simulink model "HIL_Testing_SW_amantest"  (Simulink 7.5)
settings: Solver=ode1  StartTime=0.0  StopTime=Inf  FixedStep=0.001  RelTol=1e-3
PostLoadFcn:
  | , if any(exist('dsrtsu_mdlpostloadfcn', 'file') == [2, 3, 6]), try dsrtsu_mdlpostloadfcn('Execute', bdroot); catch fprintf('Error in PostLoadFcn (dsrtsu_mdlpostloadfcn) for model "%s":\n %s\n', bdroot, lasterr); end, end,
undefined symbols (not defined in the file): CeBSER_Cnt_NumTempAxisPts, ChargeCord, ChargeCord_Control, ChargeToSOCCurr, ChrgCurrLim, CrntSens1Fine, CS_SOCSetPt, CyclerMaxChrgPwr, CyclerMaxDschrgPwr, deltaAhr, Drive_1, Drive_10, Drive_11, Drive_12, Drive_13, Drive_14, Drive_15, Drive_16, Drive_17, Drive_18, Drive_19, Drive_2, Drive_20, Drive_21, Drive_22, Drive_23, Drive_24, Drive_25, Drive_26, Drive_27, Drive_28, Drive_29, Drive_3, Drive_30, Drive_31, Drive_32, Drive_33, Drive_34, Drive_35, Drive_36, Drive_37, Drive_38, Drive_39, Drive_4, Drive_40, Drive_41, Drive_42, Drive_43, Drive_44, Drive_45, Drive_46, Drive_47, Drive_48, Drive_49, Drive_5, Drive_50, Drive_51, Drive_6, Drive_7, Drive_8 ... (+50)
libraries: simulink x129, rtican x50, rti2211sailib x5, rti2211serlib x5, rti2202miolib x3
(part 6 of 23)

== system HIL_Testing_SW_amantest/HWO/TX HVEM/msg_Charge ==
  note: unsure about this one
  HVCD_ACInputVltg : Inport  OutDataType=fixdt(1, 16)  OutScaling=2^0
  HVCD_ACInputCurr : Inport  Port=2  OutDataType=fixdt(1, 16)  OutScaling=2^0
  HVCD_ACInputTemp : Inport  Port=3  OutDataType=fixdt(1, 16)  OutScaling=2^0
  Current : Inport  Port=4  OutDataType=sfix(16)  OutScaling=2^0
  Voltage : Inport  Port=5  OutDataType=fixdt(1, 16)  OutScaling=2^0
  Trigger : TriggerPort  TriggerType=function-call
  ACInputCrntV{,1..3} (4 alike) : Constant  Value=0  OutDataTypeMode=double  OutDataType=fixdt(1, 16)  OutScaling=2^0  OutDataTypeStr=double
  ChargeFlashStat : Constant  Value=0  OutDataType=fixdt(1, 16)  OutScaling=2^0
  ChrgReadStat2 : Constant  Value=20  OutDataType=fixdt(1, 16)  OutScaling=2^0
  ChrgReadStat3 : Constant  Value=200  OutDataType=fixdt(1, 16)  OutScaling=2^0
  ChrgrPmpPrcntSpd : Constant  Value=0  OutDataType=fixdt(1, 16)  OutScaling=2^0
  HVChrgLV{,1..4} (5 alike) : Constant  OutDataType=fixdt(1, 16)  OutScaling=2^0
  High_Voltage_Charger_Data_HV : rtican/RTICAN Transmit (TX)   SystemSampleTime=-1  Reserved1=[]  Reserved2=[]  Reserved3=[]  Reserved4=[]  SfcnMessage=[]  Msg_Struct=[]  BoardTypeNo=[]  BoardNo=[]  ChannelNo=[]  Parameters=[]  DialogFcn=[]  UnitName=[]  Revision=[]  UnitValues=[]  DSProperties=struct('RTI',struct('Version',uint32(5),'BlockType',struct('isSLSource',uint8(1),'isSLSink',uint8(1),'isHWSource',uint8(0),'isHWSink',uint8(0),'isSetup',uint8(0),'isInline',uint8(1),'isNonInline',uint8(0),'isInterrupt',uint8(0),'isChannelwise',uint8(0)),'IOBoardType','RTICAN','UnitType','MESSAGE','Identifier','TX','DialogType','MSVC','BlockSet','RTICAN','SlaveProcessor','CAN'))  RTIBlockInterface=struct('InputPortsWidth',int32([1 1 1 1 1 1 1 1 1]),'InputPortsActive',[1 1 1 1 1 1 1 1 1],'InputPortsName',{{'HVChrgRdnsStat','HVCD_ChgrFlshStat','HVCD_Tmp','HVCD_ACInptVltg','HVCD_ACInptCrnt','HVCD_ACInptCrntV','HVCD_ACInptVltgV','HVCD_TmpV','HVChgrActDisStat'}},'InputPortsDataType',{{'SS_DOUBLE','SS_DOUBLE','SS_DOUBLE','SS_DOUBLE','SS_DOUBLE','SS_DOUBLE','SS_DOUBLE','SS_DOUBLE','SS_DOUBLE'}},'OutputPortsWidth',int32(1),'OutputPortsActive',1,'OutputPortsName',{{['TX status']}},'DialogFcn','rtican_message_interface_gui','BlockDisplay',{{'','center'}},'IconTransparency','on','InitLevel',3,'BlockName',struct('Token',{{'High_Voltage_Charger_Data_HV'}}),'SampleTime',{{-1}},'TriggerPort',{{'none'}},'EnablePort',{{'none'}})  RTIBlockParameters=struct('BoardTypeNo',{{4302,'OFF',[]}},'BoardNo',{{1,'ON',[1 16]}},'ChannelNo',{{4,'ON',[1 4]}},'Parameters',{{struct('DataFileSupport',struct('DataFileSelectedMaster',1,'DataFileSelectedLocal',1,'DataFileName',['c:\data\databases\8.0.1 (13015)\globala - hv.dbc|c:\data\testing\dbc\globala - hvdmx112.dbc|'],'DataFileDate',{{{['04-Jan-2013 08:37:04']},{['10-May-2011 15:46:00']}}},'SelectedFile',['..\databases\8.0.1 (13015)\globala - hv.dbc'],'InterfaceFcn','rtican_dbc_file_parser'),'Options',struct('StatusSelected',1,'TimeSelected',0,'DeltaTimeSelected',0,'DelayTimeSelected',0,'DelayTimeTXCommandSelected',0,'EncodeSetUnusedBitsToOne',0,'EnableMsgLoopback',0,'TriggerPort',struct('Selected',0,'TriggerType',0),'EnablePortSelected',0,'SignalOnPortnameSelected',1,'UserCoding',struct('Selected',0,'InterfaceFile','UserEncodingFile','FcnName','UserEncodeFcn','InportSelected',0,'InportWidth',1,'OutportSelected',0,'OutportWidth',1),'TerminationMsg',struct('Selected',0,'Byte0_7','0'),'InitialMsg',struct('Selected',0,'Byte0_7','0')),'Message',struct('MsgOnBlocknameSelected',1,'MsgName','High_Voltage_Charger_Data_HV','MsgIdFormat',0,'MsgId',778,'MsgLength',7,'NumSignals',9,'SampleTime',-1,'StartTime',struct('Selected',0,'Value',0),'AutoRepeatTime',struct('Selected',0,'Value',0.1),'Timeout',struct('Selected',0,'Value',0.1),'DelayTime',struct('Selected',0,'Value',0.1),'Signal',struct('SgnName',{'HVChrgRdnsStat','HVCD_ChgrFlshStat','HVCD_Tmp','HVCD_ACInptVltg','HVCD_ACInptCrnt','HVCD_ACInptCrntV','HVCD_ACInptVltgV','HVCD_TmpV','HVChgrActDisStat'},'SgnStartBit',{25,27,28,36,44,52,53,54,55},'SgnLength',{2,1,8,8,8,1,1,1,1},'SgnType',{0,0,0,0,0,0,0,0,0},'ModeValue',{-1,-1,-1,-1,-1,-1,-1,-1,-1},'DataType',{0,0,0,0,0,0,0,0,0},'ByteLayout',{2,2,2,2,2,2,2,2,2},'Factor',{1,1,0.5,2,0.2,1,1,1,1},'Offset',{0,0,-40,0,0,0,0,0,0},'SgnComment',{{''},{''},{''},{''},{''},{''},{''},{''},{''}},'SgnUnit',{'','',['deg C'],'V','A','','','',''},'Min',{0,0,-40,0,0,0,0,0,0},'Max',{3,1,87.5,510,51,1,1,1,1},'SLDataType',{'SS_DOUBLE','SS_DOUBLE','SS_DOUBLE','SS_DOUBLE','SS_DOUBLE','SS_DOUBLE','SS_DOUBLE','SS_DOUBLE','SS_DOUBLE'}),'MsgIdNumFormat',0,'MsgComment',{{''}}),'Version',1.2,'general',struct('isFromLib',0)),'OFF',[]}},'GroupId',{{struct('Group',{{'RTICAN'}},'No',7,'Behavior',{{'NAMECHANGE'}},'BlockType',{{'SINK'}},'NameChangeFlag',0),'OFF',[]}},'SFcnRTICANMessage',{{struct('MsgType','TX','SFcnPortType','Scalar','MsgName','High_Voltage_Charger_Data_HV','MsgIdFormat','STD','MsgId',778,'MsgLength',7,'NumSignals',9,'SampleTime',-1,'StartTime',struct('Selected','no','Value',0),'AutoRepeatTime',struct('Selected','no','Value',0.1),'Timeout',struct('Selected','no','Value',0.1),'Signal',struct('SgnName',{'HVChrgRdnsStat','HVCD_ChgrFlshStat','HVCD_Tmp','HVCD_ACInptVltg','HVCD_ACInptCrnt','HVCD_ACInptCrntV','HVCD_ACInptVltgV','HVCD_TmpV','HVChgrActDisStat'},'SgnStartBit',{25,27,28,36,44,52,53,54,55},'SgnLength',{2,1,8,8,8,1,1,1,1},'SgnType',{'standard','standard','standard','standard','standard','standard','standard','standard','standard'},'ModeValue',{-1,-1,-1,-1,-1,-1,-1,-1,-1},'DataType',{['unsigned int'],['unsigned int'],['unsigned int'],['unsigned int'],['unsigned int'],['unsigned int'],['unsigned int'],['unsigned int'],['unsigned int']},'ByteLayout',{['motorola back.'],['motorola back.'],['motorola back.'],['motorola back.'],['motorola back.'],['motorola back.'],['motorola back.'],['motorola back.'],['motorola back.']},'Factor',{1,1,0.5,2,0.2,1,1,1,1},'Offset',{0,0,-40,0,0,0,0,0,0},'SLDataType',{'SS_DOUBLE','SS_DOUBLE','SS_DOUBLE','SS_DOUBLE','SS_DOUBLE','SS_DOUBLE','SS_DOUBLE','SS_DOUBLE','SS_DOUBLE'}),'StatusSelected','yes','TimeSelected','no','DeltaTimeSelected','no','DelayTimeSelected','no','DelayTimeTXCommandSelected','no','EncodeSetUnusedBitsToOne','no','EnableMsgLoopback','no','TriggerPort',struct('Selected','no','TriggerType',0),'EnablePortSelected','no','UserCoding',struct('Selected','no','InterfaceFile','UserEncodingFile','FcnName','UserEncodeFcn','InportSelected','no','InportWidth',1,'OutportSelected','no','OutportWidth',1),'TerminationMsg',struct('Selected','no','Byte0','0x00','Byte1','0x00','Byte2','0x00','Byte3','0x00','Byte4','0x00','Byte5','0x00','Byte6','0x00','Byte7','0x00'),'InitialMsg',struct('Selected','no','Byte0','0x00','Byte1','0x00','Byte2','0x00','Byte3','0x00','Byte4','0x00','Byte5','0x00','Byte6','0x00','Byte7','0x00'),'BoardType','DS4302','BoardNo',1,'ControllerNo',4),'OFF',[]}},'TLCFileName',{{'rtican_tx_message','OFF',[]}})  RTISFcnParameters=struct('SFcnRTICANMessage','struct','TLCFileName','char')  RTIBlockParaDefault=struct('BoardTypeNo',4302,'BoardNo',1,'ChannelNo',1,'Parameters',struct('DataFileSupport',struct('DataFileSelectedMaster',0,'DataFileSelectedLocal',0,'DataFileName','','DataFileDate','','SelectedFile',['<no file selected>']),'Options',struct('StatusSelected',1,'TimeSelected',1,'DeltaTimeSelected',1,'DelayTimeSelected',1,'DelayTimeTXCommandSelected',0,'EncodeSetUnusedBitsToOne',0,'EnableMsgLoopback',0,'TriggerPort',struct('Selected',0,'TriggerType','rising'),'EnablePortSelected',0,'SignalOnPortnameSelected',1,'UserCoding',struct('Selected',0,'InterfaceFile','UserEncodingFile','FcnName','UserEncodeFcn','InportSelected',0,'InportWidth',1,'OutportSelected',0,'OutportWidth',1),'TerminationMsg',struct('Selected',0,'Byte0_7','0'),'InitialMsg',struct('Selected',0,'Byte0_7','0')),'Message',struct('MsgOnBlocknameSelected',0,'MsgName',['TX Message'],'MsgIdFormat',0,'MsgId',100,'MsgLength',8,'NumSignals',1,'SampleTime',-1,'StartTime',struct('Selected',0,'Value',0),'AutoRepeatTime',struct('Selected',0,'Value',0.1),'Timeout',struct('Selected',0,'Value',0.1),'DelayTime',struct('Selected',0,'Value',0.1),'Signal',struct('SgnName',['TX signal'],'SgnStartBit',0,'SgnLength',8,'SgnType',0,'ModeValue',-1,'DataType',0,'SLDataType','SS_DOUBLE','ByteLayout',0,'Factor',1,'Offset',0,'Min',0,'Max',255,'SgnComment',{{}},'SgnUnit',''),'MsgIdNumFormat',0,'MsgComment',{{''}}),'Version',1.2,'general',struct('isFromLib',1)),'GroupId',struct('Group',{{'RTICAN'}},'No',1,'Behavior',{{'NAMECHANGE'}},'BlockType',{{'SINK'}},'NameChangeFlag',0),'SFcnRTICANMessage',struct('MsgType','TX','MsgName',['TX Message'],'MsgIdFormat','STD','MsgId',100,'MsgLength',2,'NumSignals',1,'SampleTime',-1,'StartTime',struct('Selected','no','Value',0),'AutoRepeatTime',struct('Selected','no','Value',0.1),'Timeout',struct('Selected','no','Value',0.1),'DelayTime',struct('Selected','no','Value',0.1),'Signal',struct('SgnName',['TX signal'],'SgnStartBit',0,'SgnLength',8,'SgnType','standard','ModeValue',-1,'DataType',['unsigned int'],'ByteLayout',['little endian'],'SLDataType','SS_DOUBLE','Factor',1,'Offset',0),'StatusSelected','yes','TimeSelected','yes','DeltaTimeSelected','yes','DelayTimeSelected','yes','EnablePortSelected','no','EnableMsgLoopback','no','DelayTimeTXCommandSelected','no','EncodeSetUnusedBitsToOne','no','UserCoding',struct('Selected','no','InterfaceFile','UserDecodingFile','FcnName','UserDecodeFcn','InportSelected','no','InportWidth',1,'OutportSelected','no','OutportWidth',1),'TerminationMsg',struct('Selected','no','Byte0','0x00','Byte1','0x00','Byte2','0x00','Byte3','0x00','Byte4','0x00','Byte5','0x00','Byte6','0x00','Byte7','0x00'),'InitialMsg',struct('Selected','no','Byte0','0x00','Byte1','0x00','Byte2','0x00','Byte3','0x00','Byte4','0x00','Byte5','0x00','Byte6','0x00','Byte7','0x00'),'TriggerPort',struct('Selected','no','TriggerType','rising'),'BoardType','DS4302','BoardNo',1,'ControllerNo',1,'SFcnPortType','Scalar'),'TLCFileName','rtican_tx_message')
      settings: AttributesFormatString=Group Id: RTICAN7\n
  High_Voltage_Charger_Out_Data_HV : rtican/RTICAN Transmit (TX)   SystemSampleTime=-1  Reserved1=[]  Reserved2=[]  Reserved3=[]  Reserved4=[]  SfcnMessage=[]  Msg_Struct=[]  BoardTypeNo=[]  BoardNo=[]  ChannelNo=[]  Parameters=[]  DialogFcn=[]  UnitName=[]  Revision=[]  UnitValues=[]  DSProperties=struct('RTI',struct('Version',uint32(5),'BlockType',struct('isSLSource',uint8(1),'isSLSink',uint8(1),'isHWSource',uint8(0),'isHWSink',uint8(0),'isSetup',uint8(0),'isInline',uint8(1),'isNonInline',uint8(0),'isInterrupt',uint8(0),'isChannelwise',uint8(0)),'IOBoardType','RTICAN','UnitType','MESSAGE','Identifier','TX','DialogType','MSVC','BlockSet','RTICAN','SlaveProcessor','CAN'))  RTIBlockInterface=struct('InputPortsWidth',int32([1 1 1 1 1 1 1 1]),'InputPortsActive',[1 1 1 1 1 1 1 1],'InputPortsName',{{'HVCOD_LwVltgOptVltgV','HVCOD_LwVltgOptCrntV','HVCOD_BSOptVltgV','HVCOD_BsOptCrntV','HVCOD_LwVltgOptVltg','HVCOD_LwVltgOptCrnt','HVCOD_BSOptVltg','HVCOD_BsOptCrnt'}},'InputPortsDataType',{{'SS_DOUBLE','SS_DOUBLE','SS_DOUBLE','SS_DOUBLE','SS_DOUBLE','SS_DOUBLE','SS_DOUBLE','SS_DOUBLE'}},'OutputPortsWidth',int32(1),'OutputPortsActive',1,'OutputPortsName',{{['TX status']}},'DialogFcn','rtican_message_interface_gui','BlockDisplay',{{'','center'}},'IconTransparency','on','InitLevel',3,'BlockName',struct('Token',{{'High_Voltage_Charger_Out_Data_HV'}}),'SampleTime',{{-1}},'TriggerPort',{{'none'}},'EnablePort',{{'none'}})  RTIBlockParameters=struct('BoardTypeNo',{{4302,'OFF',[]}},'BoardNo',{{1,'ON',[1 16]}},'ChannelNo',{{4,'ON',[1 4]}},'Parameters',{{struct('DataFileSupport',struct('DataFileSelectedMaster',1,'DataFileSelectedLocal',1,'DataFileName',['c:\data\databases\8.0.1 (13015)\globala - hv.dbc|c:\data\testing\dbc\globala - hvdmx112.dbc|'],'DataFileDate',{{{['04-Jan-2013 08:37:04']},{['10-May-2011 15:46:00']}}},'SelectedFile',['..\databases\8.0.1 (13015)\globala - hv.dbc'],'InterfaceFcn','rtican_dbc_file_parser'),'Options',struct('StatusSelected',1,'TimeSelected',0,'DeltaTimeSelected',0,'DelayTimeSelected',0,'DelayTimeTXCommandSelected',0,'EncodeSetUnusedBitsToOne',0,'EnableMsgLoopback',0,'TriggerPort',struct('Selected',0,'TriggerType',0),'EnablePortSelected',0,'SignalOnPortnameSelected',1,'UserCoding',struct('Selected',0,'InterfaceFile','UserEncodingFile','FcnName','UserEncodeFcn','InportSelected',0,'InportWidth',1,'OutportSelected',0,'OutportWidth',1),'TerminationMsg',struct('Selected',0,'Byte0_7','0'),'InitialMsg',struct('Selected',0,'Byte0_7','0')),'Message',struct('MsgOnBlocknameSelected',1,'MsgName','High_Voltage_Charger_Out_Data_HV','MsgIdFormat',0,'MsgId',530,'MsgLength',6,'NumSignals',8,'SampleTime',-1,'StartTime',struct('Selected',0,'Value',0),'AutoRepeatTime',struct('Selected',0,'Value',0.1),'Timeout',struct('Selected',0,'Value',0.1),'DelayTime',struct('Selected',0,'Value',0.1),'Signal',struct('SgnName',{'HVCOD_LwVltgOptVltgV','HVCOD_LwVltgOptCrntV','HVCOD_BSOptVltgV','HVCOD_BsOptCrntV','HVCOD_LwVltgOptVltg','HVCOD_LwVltgOptCrnt','HVCOD_BSOptVltg','HVCOD_BsOptCrnt'},'SgnStartBit',{5,6,7,8,9,17,25,35},'SgnLength',{1,1,1,1,8,8,10,10},'SgnType',{0,0,0,0,0,0,0,0},'ModeValue',{-1,-1,-1,-1,-1,-1,-1,-1},'DataType',{0,0,0,0,0,0,0,0},'ByteLayout',{2,2,2,2,2,2,2,2},'Factor',{1,1,1,1,0.1,0.2,0.5,0.05},'Offset',{0,0,0,0,0,0,0,0},'SgnComment',{{''},{''},{''},{''},{''},{''},{''},{''}},'SgnUnit',{'','','','','V','A','V','A'},'Min',{0,0,0,0,0,0,0,0},'Max',{1,1,1,1,25.5,51,511.5,51.15},'SLDataType',{'SS_DOUBLE','SS_DOUBLE','SS_DOUBLE','SS_DOUBLE','SS_DOUBLE','SS_DOUBLE','SS_DOUBLE','SS_DOUBLE'}),'MsgIdNumFormat',1,'MsgComment',{{''}}),'Version',1.2,'general',struct('isFromLib',0)),'OFF',[]}},'GroupId',{{struct('Group',{{'RTICAN'}},'No',7,'Behavior',{{'NAMECHANGE'}},'BlockType',{{'SINK'}},'NameChangeFlag',0),'OFF',[]}},'SFcnRTICANMessage',{{struct('MsgType','TX','SFcnPortType','Scalar','MsgName','High_Voltage_Charger_Out_Data_HV','MsgIdFormat','STD','MsgId',530,'MsgLength',6,'NumSignals',8,'SampleTime',-1,'StartTime',struct('Selected','no','Value',0),'AutoRepeatTime',struct('Selected','no','Value',0.1),'Timeout',struct('Selected','no','Value',0.1),'Signal',struct('SgnName',{'HVCOD_LwVltgOptVltgV','HVCOD_LwVltgOptCrntV','HVCOD_BSOptVltgV','HVCOD_BsOptCrntV','HVCOD_LwVltgOptVltg','HVCOD_LwVltgOptCrnt','HVCOD_BSOptVltg','HVCOD_BsOptCrnt'},'SgnStartBit',{5,6,7,8,9,17,25,35},'SgnLength',{1,1,1,1,8,8,10,10},'SgnType',{'standard','standard','standard','standard','standard','standard','standard','standard'},'ModeValue',{-1,-1,-1,-1,-1,-1,-1,-1},'DataType',{['unsigned int'],['unsigned int'],['unsigned int'],['unsigned int'],['unsigned int'],['unsigned int'],['unsigned int'],['unsigned int']},'ByteLayout',{['motorola back.'],['motorola back.'],['motorola back.'],['motorola back.'],['motorola back.'],['motorola back.'],['motorola back.'],['motorola back.']},'Factor',{1,1,1,1,0.1,0.2,0.5,0.05},'Offset',{0,0,0,0,0,0,0,0},'SLDataType',{'SS_DOUBLE','SS_DOUBLE','SS_DOUBLE','SS_DOUBLE','SS_DOUBLE','SS_DOUBLE','SS_DOUBLE','SS_DOUBLE'}),'StatusSelected','yes','TimeSelected','no','DeltaTimeSelected','no','DelayTimeSelected','no','DelayTimeTXCommandSelected','no','EncodeSetUnusedBitsToOne','no','EnableMsgLoopback','no','TriggerPort',struct('Selected','no','TriggerType',0),'EnablePortSelected','no','UserCoding',struct('Selected','no','InterfaceFile','UserEncodingFile','FcnName','UserEncodeFcn','InportSelected','no','InportWidth',1,'OutportSelected','no','OutportWidth',1),'TerminationMsg',struct('Selected','no','Byte0','0x00','Byte1','0x00','Byte2','0x00','Byte3','0x00','Byte4','0x00','Byte5','0x00','Byte6','0x00','Byte7','0x00'),'InitialMsg',struct('Selected','no','Byte0','0x00','Byte1','0x00','Byte2','0x00','Byte3','0x00','Byte4','0x00','Byte5','0x00','Byte6','0x00','Byte7','0x00'),'BoardType','DS4302','BoardNo',1,'ControllerNo',4),'OFF',[]}},'TLCFileName',{{'rtican_tx_message','OFF',[]}})  RTISFcnParameters=struct('SFcnRTICANMessage','struct','TLCFileName','char')  RTIBlockParaDefault=struct('BoardTypeNo',4302,'BoardNo',1,'ChannelNo',1,'Parameters',struct('DataFileSupport',struct('DataFileSelectedMaster',0,'DataFileSelectedLocal',0,'DataFileName','','DataFileDate','','SelectedFile',['<no file selected>']),'Options',struct('StatusSelected',1,'TimeSelected',1,'DeltaTimeSelected',1,'DelayTimeSelected',1,'DelayTimeTXCommandSelected',0,'EncodeSetUnusedBitsToOne',0,'EnableMsgLoopback',0,'TriggerPort',struct('Selected',0,'TriggerType','rising'),'EnablePortSelected',0,'SignalOnPortnameSelected',1,'UserCoding',struct('Selected',0,'InterfaceFile','UserEncodingFile','FcnName','UserEncodeFcn','InportSelected',0,'InportWidth',1,'OutportSelected',0,'OutportWidth',1),'TerminationMsg',struct('Selected',0,'Byte0_7','0'),'InitialMsg',struct('Selected',0,'Byte0_7','0')),'Message',struct('MsgOnBlocknameSelected',0,'MsgName',['TX Message'],'MsgIdFormat',0,'MsgId',100,'MsgLength',8,'NumSignals',1,'SampleTime',-1,'StartTime',struct('Selected',0,'Value',0),'AutoRepeatTime',struct('Selected',0,'Value',0.1),'Timeout',struct('Selected',0,'Value',0.1),'DelayTime',struct('Selected',0,'Value',0.1),'Signal',struct('SgnName',['TX signal'],'SgnStartBit',0,'SgnLength',8,'SgnType',0,'ModeValue',-1,'DataType',0,'SLDataType','SS_DOUBLE','ByteLayout',0,'Factor',1,'Offset',0,'Min',0,'Max',255,'SgnComment',{{}},'SgnUnit',''),'MsgIdNumFormat',0,'MsgComment',{{''}}),'Version',1.2,'general',struct('isFromLib',1)),'GroupId',struct('Group',{{'RTICAN'}},'No',1,'Behavior',{{'NAMECHANGE'}},'BlockType',{{'SINK'}},'NameChangeFlag',0),'SFcnRTICANMessage',struct('MsgType','TX','MsgName',['TX Message'],'MsgIdFormat','STD','MsgId',100,'MsgLength',2,'NumSignals',1,'SampleTime',-1,'StartTime',struct('Selected','no','Value',0),'AutoRepeatTime',struct('Selected','no','Value',0.1),'Timeout',struct('Selected','no','Value',0.1),'DelayTime',struct('Selected','no','Value',0.1),'Signal',struct('SgnName',['TX signal'],'SgnStartBit',0,'SgnLength',8,'SgnType','standard','ModeValue',-1,'DataType',['unsigned int'],'ByteLayout',['little endian'],'SLDataType','SS_DOUBLE','Factor',1,'Offset',0),'StatusSelected','yes','TimeSelected','yes','DeltaTimeSelected','yes','DelayTimeSelected','yes','EnablePortSelected','no','EnableMsgLoopback','no','DelayTimeTXCommandSelected','no','EncodeSetUnusedBitsToOne','no','UserCoding',struct('Selected','no','InterfaceFile','UserDecodingFile','FcnName','UserDecodeFcn','InportSelected','no','InportWidth',1,'OutportSelected','no','OutportWidth',1),'TerminationMsg',struct('Selected','no','Byte0','0x00','Byte1','0x00','Byte2','0x00','Byte3','0x00','Byte4','0x00','Byte5','0x00','Byte6','0x00','Byte7','0x00'),'InitialMsg',struct('Selected','no','Byte0','0x00','Byte1','0x00','Byte2','0x00','Byte3','0x00','Byte4','0x00','Byte5','0x00','Byte6','0x00','Byte7','0x00'),'TriggerPort',struct('Selected','no','TriggerType','rising'),'BoardType','DS4302','BoardNo',1,'ControllerNo',1,'SFcnPortType','Scalar'),'TLCFileName','rtican_tx_message')
      settings: AttributesFormatString=Group Id: RTICAN7\n
  High_Voltage_Charger_info_2_HV : rtican/RTICAN Transmit (TX)   SystemSampleTime=-1  Reserved1=[]  Reserved2=[]  Reserved3=[]  Reserved4=[]  SfcnMessage=[]  Msg_Struct=[]  BoardTypeNo=[]  BoardNo=[]  ChannelNo=[]  Parameters=[]  DialogFcn=[]  UnitName=[]  Revision=[]  UnitValues=[]  DSProperties=struct('RTI',struct('Version',uint32(5),'BlockType',struct('isSLSource',uint8(1),'isSLSink',uint8(1),'isHWSource',uint8(0),'isHWSink',uint8(0),'isSetup',uint8(0),'isInline',uint8(1),'isNonInline',uint8(0),'isInterrupt',uint8(0),'isChannelwise',uint8(0)),'IOBoardType','RTICAN','UnitType','MESSAGE','Identifier','TX','DialogType','MSVC','BlockSet','RTICAN','SlaveProcessor','CAN'))  RTIBlockInterface=struct('InputPortsWidth',int32([1 1 1 1]),'InputPortsActive',[1 1 1 1],'InputPortsName',{{'HVChrgrLVPwrSplyStat','HVChrgr12VWkStat','HVChrgrHVPwrSplyStat','HVChrgrPFCPwrSplyStat'}},'InputPortsDataType',{{'SS_DOUBLE','SS_DOUBLE','SS_DOUBLE','SS_DOUBLE'}},'OutputPortsWidth',int32(1),'OutputPortsActive',1,'OutputPortsName',{{['TX status']}},'DialogFcn','rtican_message_interface_gui','BlockDisplay',{{'','center'}},'IconTransparency','on','InitLevel',3,'BlockName',struct('Token',{{'High_Voltage_Charger_info_2_HV'}}),'SampleTime',{{-1}},'TriggerPort',{{'none'}},'EnablePort',{{'none'}})  RTIBlockParameters=struct('BoardTypeNo',{{4302,'OFF',[]}},'BoardNo',{{1,'ON',[1 16]}},'ChannelNo',{{4,'ON',[1 4]}},'Parameters',{{struct('DataFileSupport',struct('DataFileSelectedMaster',1,'DataFileSelectedLocal',1,'DataFileName',['c:\data\databases\8.0.1 (13015)\globala - hv.dbc|c:\data\testing\dbc\globala - hvdmx112.dbc|'],'DataFileDate',{{{['04-Jan-2013 08:37:04']},{['10-May-2011 15:46:00']}}},'SelectedFile',['..\databases\8.0.1 (13015)\globala - hv.dbc'],'InterfaceFcn','rtican_dbc_file_parser'),'Options',struct('StatusSelected',1,'TimeSelected',0,'DeltaTimeSelected',0,'DelayTimeSelected',0,'DelayTimeTXCommandSelected',0,'EncodeSetUnusedBitsToOne',0,'EnableMsgLoopback',0,'TriggerPort',struct('Selected',0,'TriggerType',0),'EnablePortSelected',0,'SignalOnPortnameSelected',1,'UserCoding',struct('Selected',0,'InterfaceFile','UserEncodingFile','FcnName','UserEncodeFcn','InportSelected',0,'InportWidth',1,'OutportSelected',0,'OutportWidth',1),'TerminationMsg',struct('Selected',0,'Byte0_7','0'),'InitialMsg',struct('Selected',0,'Byte0_7','0')),'Message',struct('MsgOnBlocknameSelected',1,'MsgName','High_Voltage_Charger_info_2_HV','MsgIdFormat',0,'MsgId',776,'MsgLength',5,'NumSignals',4,'SampleTime',-1,'StartTime',struct('Selected',0,'Value',0),'AutoRepeatTime',struct('Selected',0,'Value',0.1),'Timeout',struct('Selected',0,'Value',0.1),'DelayTime',struct('Selected',0,'Value',0.1),'Signal',struct('SgnName',{'HVChrgrLVPwrSplyStat','HVChrgr12VWkStat','HVChrgrHVPwrSplyStat','HVChrgrPFCPwrSplyStat'},'SgnStartBit',{19,20,21,22},'SgnLength',{1,1,1,1},'SgnType',{0,0,0,0},'ModeValue',{-1,-1,-1,-1},'DataType',{0,0,0,0},'ByteLayout',{2,2,2,2},'Factor',{1,1,1,1},'Offset',{0,0,0,0},'SgnComment',{{''},{''},{''},{''}},'SgnUnit',{'','','',''},'Min',{0,0,0,0},'Max',{1,1,1,1},'SLDataType',{'SS_DOUBLE','SS_DOUBLE','SS_DOUBLE','SS_DOUBLE'}),'MsgIdNumFormat',1,'MsgComment',{{''}}),'Version',1.2,'general',struct('isFromLib',0)),'OFF',[]}},'GroupId',{{struct('Group',{{'RTICAN'}},'No',7,'Behavior',{{'NAMECHANGE'}},'BlockType',{{'SINK'}},'NameChangeFlag',0),'OFF',[]}},'SFcnRTICANMessage',{{struct('MsgType','TX','SFcnPortType','Scalar','MsgName','High_Voltage_Charger_info_2_HV','MsgIdFormat','STD','MsgId',776,'MsgLength',5,'NumSignals',4,'SampleTime',-1,'StartTime',struct('Selected','no','Value',0),'AutoRepeatTime',struct('Selected','no','Value',0.1),'Timeout',struct('Selected','no','Value',0.1),'Signal',struct('SgnName',{'HVChrgrLVPwrSplyStat','HVChrgr12VWkStat','HVChrgrHVPwrSplyStat','HVChrgrPFCPwrSplyStat'},'SgnStartBit',{19,20,21,22},'SgnLength',{1,1,1,1},'SgnType',{'standard','standard','standard','standard'},'ModeValue',{-1,-1,-1,-1},'DataType',{['unsigned int'],['unsigned int'],['unsigned int'],['unsigned int']},'ByteLayout',{['motorola back.'],['motorola back.'],['motorola back.'],['motorola back.']},'Factor',{1,1,1,1},'Offset',{0,0,0,0},'SLDataType',{'SS_DOUBLE','SS_DOUBLE','SS_DOUBLE','SS_DOUBLE'}),'StatusSelected','yes','TimeSelected','no','DeltaTimeSelected','no','DelayTimeSelected','no','DelayTimeTXCommandSelected','no','EncodeSetUnusedBitsToOne','no','EnableMsgLoopback','no','TriggerPort',struct('Selected','no','TriggerType',0),'EnablePortSelected','no','UserCoding',struct('Selected','no','InterfaceFile','UserEncodingFile','FcnName','UserEncodeFcn','InportSelected','no','InportWidth',1,'OutportSelected','no','OutportWidth',1),'TerminationMsg',struct('Selected','no','Byte0','0x00','Byte1','0x00','Byte2','0x00','Byte3','0x00','Byte4','0x00','Byte5','0x00','Byte6','0x00','Byte7','0x00'),'InitialMsg',struct('Selected','no','Byte0','0x00','Byte1','0x00','Byte2','0x00','Byte3','0x00','Byte4','0x00','Byte5','0x00','Byte6','0x00','Byte7','0x00'),'BoardType','DS4302','BoardNo',1,'ControllerNo',4),'OFF',[]}},'TLCFileName',{{'rtican_tx_message','OFF',[]}})  RTISFcnParameters=struct('SFcnRTICANMessage','struct','TLCFileName','char')  RTIBlockParaDefault=struct('BoardTypeNo',4302,'BoardNo',1,'ChannelNo',1,'Parameters',struct('DataFileSupport',struct('DataFileSelectedMaster',0,'DataFileSelectedLocal',0,'DataFileName','','DataFileDate','','SelectedFile',['<no file selected>']),'Options',struct('StatusSelected',1,'TimeSelected',1,'DeltaTimeSelected',1,'DelayTimeSelected',1,'DelayTimeTXCommandSelected',0,'EncodeSetUnusedBitsToOne',0,'EnableMsgLoopback',0,'TriggerPort',struct('Selected',0,'TriggerType','rising'),'EnablePortSelected',0,'SignalOnPortnameSelected',1,'UserCoding',struct('Selected',0,'InterfaceFile','UserEncodingFile','FcnName','UserEncodeFcn','InportSelected',0,'InportWidth',1,'OutportSelected',0,'OutportWidth',1),'TerminationMsg',struct('Selected',0,'Byte0_7','0'),'InitialMsg',struct('Selected',0,'Byte0_7','0')),'Message',struct('MsgOnBlocknameSelected',0,'MsgName',['TX Message'],'MsgIdFormat',0,'MsgId',100,'MsgLength',8,'NumSignals',1,'SampleTime',-1,'StartTime',struct('Selected',0,'Value',0),'AutoRepeatTime',struct('Selected',0,'Value',0.1),'Timeout',struct('Selected',0,'Value',0.1),'DelayTime',struct('Selected',0,'Value',0.1),'Signal',struct('SgnName',['TX signal'],'SgnStartBit',0,'SgnLength',8,'SgnType',0,'ModeValue',-1,'DataType',0,'SLDataType','SS_DOUBLE','ByteLayout',0,'Factor',1,'Offset',0,'Min',0,'Max',255,'SgnComment',{{}},'SgnUnit',''),'MsgIdNumFormat',0,'MsgComment',{{''}}),'Version',1.2,'general',struct('isFromLib',1)),'GroupId',struct('Group',{{'RTICAN'}},'No',1,'Behavior',{{'NAMECHANGE'}},'BlockType',{{'SINK'}},'NameChangeFlag',0),'SFcnRTICANMessage',struct('MsgType','TX','MsgName',['TX Message'],'MsgIdFormat','STD','MsgId',100,'MsgLength',2,'NumSignals',1,'SampleTime',-1,'StartTime',struct('Selected','no','Value',0),'AutoRepeatTime',struct('Selected','no','Value',0.1),'Timeout',struct('Selected','no','Value',0.1),'DelayTime',struct('Selected','no','Value',0.1),'Signal',struct('SgnName',['TX signal'],'SgnStartBit',0,'SgnLength',8,'SgnType','standard','ModeValue',-1,'DataType',['unsigned int'],'ByteLayout',['little endian'],'SLDataType','SS_DOUBLE','Factor',1,'Offset',0),'StatusSelected','yes','TimeSelected','yes','DeltaTimeSelected','yes','DelayTimeSelected','yes','EnablePortSelected','no','EnableMsgLoopback','no','DelayTimeTXCommandSelected','no','EncodeSetUnusedBitsToOne','no','UserCoding',struct('Selected','no','InterfaceFile','UserDecodingFile','FcnName','UserDecodeFcn','InportSelected','no','InportWidth',1,'OutportSelected','no','OutportWidth',1),'TerminationMsg',struct('Selected','no','Byte0','0x00','Byte1','0x00','Byte2','0x00','Byte3','0x00','Byte4','0x00','Byte5','0x00','Byte6','0x00','Byte7','0x00'),'InitialMsg',struct('Selected','no','Byte0','0x00','Byte1','0x00','Byte2','0x00','Byte3','0x00','Byte4','0x00','Byte5','0x00','Byte6','0x00','Byte7','0x00'),'TriggerPort',struct('Selected','no','TriggerType','rising'),'BoardType','DS4302','BoardNo',1,'ControllerNo',1,'SFcnPortType','Scalar'),'TLCFileName','rtican_tx_message')
      settings: AttributesFormatString=Group Id: RTICAN7\n
  PPEI_Trans_General_Status_2 : rtican/RTICAN Transmit (TX)   SystemSampleTime=-1  Reserved1=[]  Reserved2=[]  Reserved3=[]  Reserved4=[]  SfcnMessage=[]  Msg_Struct=[]  BoardTypeNo=[]  BoardNo=[]  ChannelNo=[]  Parameters=[]  DialogFcn=[]  UnitName=[]  Revision=[]  UnitValues=[]  DSProperties=struct('RTI',struct('Version',uint32(5),'BlockType',struct('isSLSource',uint8(1),'isSLSink',uint8(1),'isHWSource',uint8(0),'isHWSink',uint8(0),'isSetup',uint8(0),'isInline',uint8(1),'isNonInline',uint8(0),'isInterrupt',uint8(0),'isChannelwise',uint8(0)),'IOBoardType','RTICAN','UnitType','MESSAGE','Identifier','TX','DialogType','MSVC','BlockSet','RTICAN','SlaveProcessor','CAN'))  RTIBlockInterface=struct('InputPortsWidth',int32([1 1 1 1 1 1 1 1 1 1 1 1 1 1 1 1 1 1 1 1 1 1 1 1 1 1 1 1 1]),'InputPortsActive',[1 1 1 1 1 1 1 1 1 1 1 1 1 1 1 1 1 1 1 1 1 1 1 1 1 1 1 1 1],'InputPortsName',{{'CltchPdlActPos','TrnsEngdState','TrnsEngdStateV','TrnsFldPrsPrsnt','TrnsPattSelEcnMdOCm','EngRecDwnshftIO','CltchPdlActPosV','TransTUDMdStat','TrnShftPtrnActStat','TmpDrvrShftCtlAct','TrnCrpMdAtv','TrnsShftLvrLckRqd','TrnsSftMdStat','CltStartSwAtv','CltStartSwAtvV','TrnsShftLvrPos','TrnsShftLvrPosV','TrnsRngInhbtStat','DrvtShftCntrlTrgtGear','DrShftCntrlReqDndIO','EngRecmndUpshftIO','TrnsSkpShftIO','AutoTransComndGear','AutoTransGrSftDirect','TopTrvlCltchSwAct','TopTrvlCltchSwActV','TransEstGear','TransEstGearV','TrnsTrqCnvCltCmndMd'}},'InputPortsDataType',{{'SS_DOUBLE','SS_DOUBLE','SS_DOUBLE','SS_DOUBLE','SS_DOUBLE','SS_DOUBLE','SS_DOUBLE','SS_DOUBLE','SS_DOUBLE','SS_DOUBLE','SS_DOUBLE','SS_DOUBLE','SS_DOUBLE','SS_DOUBLE','SS_DOUBLE','SS_DOUBLE','SS_DOUBLE','SS_DOUBLE','SS_DOUBLE','SS_DOUBLE','SS_DOUBLE','SS_DOUBLE','SS_DOUBLE','SS_DOUBLE','SS_DOUBLE','SS_DOUBLE','SS_DOUBLE','SS_DOUBLE','SS_DOUBLE'}},'OutputPortsWidth',int32(1),'OutputPortsActive',1,'OutputPortsName',{{['TX status']}},'DialogFcn','rtican_message_interface_gui','BlockDisplay',{{'','center'}},'IconTransparency','on','InitLevel',3,'BlockName',struct('Token',{{'PPEI_Trans_General_Status_2'}}),'SampleTime',{{-1}},'TriggerPort',{{'none'}},'EnablePort',{{'none'}})  RTIBlockParameters=struct('BoardTypeNo',{{4302,'OFF',[]}},'BoardNo',{{1,'ON',[1 16]}},'ChannelNo',{{1,'ON',[1 4]}},'Parameters',{{struct('DataFileSupport',struct('DataFileSelectedMaster',1,'DataFileSelectedLocal',1,'DataFileName',['c:\data\databases\8.4.5 (140425)\globala - hs.dbc|'],'DataFileDate',['24-Apr-2014 15:37:04'],'SelectedFile',['..\databases\8.4.5 (140425)\globala - hs.dbc'],'InterfaceFcn','rtican_dbc_file_parser'),'Options',struct('StatusSelected',1,'TimeSelected',0,'DeltaTimeSelected',0,'DelayTimeSelected',0,'DelayTimeTXCommandSelected',0,'EncodeSetUnusedBitsToOne',0,'EnableMsgLoopback',0,'TriggerPort',struct('Selected',0,'TriggerType',0),'EnablePortSelected',0,'SignalOnPortnameSelected',1,'UserCoding',struct('Selected',0,'InterfaceFile','UserEncodingFile','FcnName','UserEncodeFcn','InportSelected',0,'InportWidth',1,'OutportSelected',0,'OutportWidth',1),'TerminationMsg',struct('Selected',0,'Byte0_7','0'),'InitialMsg',struct('Selected',0,'Byte0_7','0')),'Message',struct('MsgOnBlocknameSelected',1,'MsgName','PPEI_Trans_General_Status_2','MsgIdFormat',0,'MsgId',501,'MsgLength',8,'NumSignals',29,'SampleTime',-1,'StartTime',struct('Selected',0,'Value',0),'AutoRepeatTime',struct('Selected',0,'Value',0.1),'Timeout',struct('Selected',0,'Value',0.1),'DelayTime',struct('Selected',0,'Value',0.1),'Signal',struct('SgnName',{'CltchPdlActPos','TrnsEngdState','TrnsEngdStateV','TrnsFldPrsPrsnt','TrnsPattSelEcnMdOCm','EngRecDwnshftIO','CltchPdlActPosV','TransTUDMdStat','TrnShftPtrnActStat','TmpDrvrShftCtlAct','TrnCrpMdAtv','TrnsShftLvrLckRqd','TrnsSftMdStat','CltStartSwAtv','CltStartSwAtvV','TrnsShftLvrPos','TrnsShftLvrPosV','TrnsRngInhbtStat','DrvtShftCntrlTrgtGear','DrShftCntrlReqDndIO','EngRecmndUpshftIO','TrnsSkpShftIO','AutoTransComndGear','AutoTransGrSftDirect','TopTrvlCltchSwAct','TopTrvlCltchSwActV','TransEstGear','TransEstGearV','TrnsTrqCnvCltCmndMd'},'SgnStartBit',{0,8,10,11,12,14,15,16,18,21,22,23,24,29,30,32,36,37,40,45,46,47,48,52,54,55,56,60,61},'SgnLength',{8,2,1,1,1,1,1,2,3,1,1,1,3,1,1,4,1,3,4,1,1,1,4,2,1,1,4,1,3},'SgnType',{0,0,0,0,0,0,0,0,0,0,0,0,0,0,0,0,0,0,0,0,0,0,0,0,0,0,0,0,0},'ModeValue',{-1,-1,-1,-1,-1,-1,-1,-1,-1,-1,-1,-1,-1,-1,-1,-1,-1,-1,-1,-1,-1,-1,-1,-1,-1,-1,-1,-1,-1},'DataType',{0,0,0,0,0,0,0,0,0,0,0,0,0,0,0,0,0,0,0,0,0,0,0,0,0,0,0,0,0},'ByteLayout',{2,2,2,2,2,2,2,2,2,2,2,2,2,2,2,2,2,2,2,2,2,2,2,2,2,2,2,2,2},'Factor',{0.392157,1,1,1,1,1,1,1,1,1,1,1,1,1,1,1,1,1,1,1,1,1,1,1,1,1,1,1,1},'Offset',{0,0,0,0,0,0,0,0,0,0,0,0,0,0,0,0,0,0,0,0,0,0,0,0,0,0,0,0,0},'SgnComment',{{''},{''},{''},{''},{''},{''},{''},{''},{['(PT = Powertrain)']},{''},{''},{''},{''},{''},{''},{''},{''},{''},{''},{''},{''},{''},{''},{''},{''},{''},{''},{''},{''}},'SgnUnit',{'%','','','','','','','','','','','','','','','','','','','','','','','','','','','',''},'Min',{0,0,0,0,0,0,0,0,0,0,0,0,0,0,0,0,0,0,0,0,0,0,0,0,0,0,0,0,0},'Max',{100.000035,3,1,1,1,1,1,3,7,1,1,1,7,1,1,15,1,7,15,1,1,1,15,3,1,1,15,1,7},'SLDataType',{'SS_DOUBLE','SS_DOUBLE','SS_DOUBLE','SS_DOUBLE','SS_DOUBLE','SS_DOUBLE','SS_DOUBLE','SS_DOUBLE','SS_DOUBLE','SS_DOUBLE','SS_DOUBLE','SS_DOUBLE','SS_DOUBLE','SS_DOUBLE','SS_DOUBLE','SS_DOUBLE','SS_DOUBLE','SS_DOUBLE','SS_DOUBLE','SS_DOUBLE','SS_DOUBLE','SS_DOUBLE','SS_DOUBLE','SS_DOUBLE','SS_DOUBLE','SS_DOUBLE','SS_DOUBLE','SS_DOUBLE','SS_DOUBLE'}),'MsgIdNumFormat',1,'MsgComment',{{''}}),'Version',1.2,'general',struct('isFromLib',0)),'OFF',[]}},'GroupId',{{struct('Group',{{'RTICAN'}},'No',8,'Behavior',{{'NAMECHANGE'}},'BlockType',{{'SINK'}},'NameChangeFlag',0),'OFF',[]}},'SFcnRTICANMessage',{{struct('MsgType','TX','SFcnPortType','Scalar','MsgName','PPEI_Trans_General_Status_2','MsgIdFormat','STD','MsgId',501,'MsgLength',8,'NumSignals',29,'SampleTime',-1,'StartTime',struct('Selected','no','Value',0),'AutoRepeatTime',struct('Selected','no','Value',0.1),'Timeout',struct('Selected','no','Value',0.1),'Signal',struct('SgnName',{'CltchPdlActPos','TrnsEngdState','TrnsEngdStateV','TrnsFldPrsPrsnt','TrnsPattSelEcnMdOCm','EngRecDwnshftIO','CltchPdlActPosV','TransTUDMdStat','TrnShftPtrnActStat','TmpDrvrShftCtlAct','TrnCrpMdAtv','TrnsShftLvrLckRqd','TrnsSftMdStat','CltStartSwAtv','CltStartSwAtvV','TrnsShftLvrPos','TrnsShftLvrPosV','TrnsRngInhbtStat','DrvtShftCntrlTrgtGear','DrShftCntrlReqDndIO','EngRecmndUpshftIO','TrnsSkpShftIO','AutoTransComndGear','AutoTransGrSftDirect','TopTrvlCltchSwAct','TopTrvlCltchSwActV','TransEstGear','TransEstGearV','TrnsTrqCnvCltCmndMd'},'SgnStartBit',{0,8,10,11,12,14,15,16,18,21,22,23,24,29,30,32,36,37,40,45,46,47,48,52,54,55,56,60,61},'SgnLength',{8,2,1,1,1,1,1,2,3,1,1,1,3,1,1,4,1,3,4,1,1,1,4,2,1,1,4,1,3},'SgnType',{'standard','standard','standard','standard','standard','standard','standard','standard','standard','standard','standard','standard','standard','standard','standard','standard','standard','standard','standard','standard','standard','standard','standard','standard','standard','standard','standard','standard','standard'},'ModeValue',{-1,-1,-1,-1,-1,-1,-1,-1,-1,-1,-1,-1,-1,-1,-1,-1,-1,-1,-1,-1,-1,-1,-1,-1,-1,-1,-1,-1,-1},'DataType',{['unsigned int'],['unsigned int'],['unsigned int'],['unsigned int'],['unsigned int'],['unsigned int'],['unsigned int'],['unsigned int'],['unsigned int'],['unsigned int'],['unsigned int'],['unsigned int'],['unsigned int'],['unsigned int'],['unsigned int'],['unsigned int'],['unsigned int'],['unsigned int'],['unsigned int'],['unsigned int'],['unsigned int'],['unsigned int'],['unsigned int'],['unsigned int'],['unsigned int'],['unsigned int'],['unsigned int'],['unsigned int'],['unsigned int']},'ByteLayout',{['motorola back.'],['motorola back.'],['motorola back.'],['motorola back.'],['motorola back.'],['motorola back.'],['motorola back.'],['motorola back.'],['motorola back.'],['motorola back.'],['motorola back.'],['motorola back.'],['motorola back.'],['motorola back.'],['motorola back.'],['motorola back.'],['motorola back.'],['motorola back.'],['motorola back.'],['motorola back.'],['motorola back.'],['motorola back.'],['motorola back.'],['motorola back.'],['motorola back.'],['motorola back.'],['motorola back.'],['motorola back.'],['motorola back.']},'Factor',{0.392157,1,1,1,1,1,1,1,1,1,1,1,1,1,1,1,1,1,1,1,1,1,1,1,1,1,1,1,1},'Offset',{0,0,0,0,0,0,0,0,0,0,0,0,0,0,0,0,0,0,0,0,0,0,0,0,0,0,0,0,0},'SLDataType',{'SS_DOUBLE','SS_DOUBLE','SS_DOUBLE','SS_DOUBLE','SS_DOUBLE','SS_DOUBLE','SS_DOUBLE','SS_DOUBLE','SS_DOUBLE','SS_DOUBLE','SS_DOUBLE','SS_DOUBLE','SS_DOUBLE','SS_DOUBLE','SS_DOUBLE','SS_DOUBLE','SS_DOUBLE','SS_DOUBLE','SS_DOUBLE','SS_DOUBLE','SS_DOUBLE','SS_DOUBLE','SS_DOUBLE','SS_DOUBLE','SS_DOUBLE','SS_DOUBLE','SS_DOUBLE','SS_DOUBLE','SS_DOUBLE'}),'StatusSelected','yes','TimeSelected','no','DeltaTimeSelected','no','DelayTimeSelected','no','DelayTimeTXCommandSelected','no','EncodeSetUnusedBitsToOne','no','EnableMsgLoopback','no','TriggerPort',struct('Selected','no','TriggerType',0),'EnablePortSelected','no','UserCoding',struct('Selected','no','InterfaceFile','UserEncodingFile','FcnName','UserEncodeFcn','InportSelected','no','InportWidth',1,'OutportSelected','no','OutportWidth',1),'TerminationMsg',struct('Selected','no','Byte0','0x00','Byte1','0x00','Byte2','0x00','Byte3','0x00','Byte4','0x00','Byte5','0x00','Byte6','0x00','Byte7','0x00'),'InitialMsg',struct('Selected','no','Byte0','0x00','Byte1','0x00','Byte2','0x00','Byte3','0x00','Byte4','0x00','Byte5','0x00','Byte6','0x00','Byte7','0x00'),'BoardType','DS4302','BoardNo',1,'ControllerNo',1),'OFF',[]}},'TLCFileName',{{'rtican_tx_message','OFF',[]}})  RTISFcnParameters=struct('SFcnRTICANMessage','struct','TLCFileName','char')  RTIBlockParaDefault=struct('BoardTypeNo',4302,'BoardNo',1,'ChannelNo',1,'Parameters',struct('DataFileSupport',struct('DataFileSelectedMaster',0,'DataFileSelectedLocal',0,'DataFileName','','DataFileDate','','SelectedFile',['<no file selected>']),'Options',struct('StatusSelected',1,'TimeSelected',1,'DeltaTimeSelected',1,'DelayTimeSelected',1,'DelayTimeTXCommandSelected',0,'EncodeSetUnusedBitsToOne',0,'EnableMsgLoopback',0,'TriggerPort',struct('Selected',0,'TriggerType','rising'),'EnablePortSelected',0,'SignalOnPortnameSelected',1,'UserCoding',struct('Selected',0,'InterfaceFile','UserEncodingFile','FcnName','UserEncodeFcn','InportSelected',0,'InportWidth',1,'OutportSelected',0,'OutportWidth',1),'TerminationMsg',struct('Selected',0,'Byte0_7','0'),'InitialMsg',struct('Selected',0,'Byte0_7','0')),'Message',struct('MsgOnBlocknameSelected',0,'MsgName',['TX Message'],'MsgIdFormat',0,'MsgId',100,'MsgLength',8,'NumSignals',1,'SampleTime',-1,'StartTime',struct('Selected',0,'Value',0),'AutoRepeatTime',struct('Selected',0,'Value',0.1),'Timeout',struct('Selected',0,'Value',0.1),'DelayTime',struct('Selected',0,'Value',0.1),'Signal',struct('SgnName',['TX signal'],'SgnStartBit',0,'SgnLength',8,'SgnType',0,'ModeValue',-1,'DataType',0,'SLDataType','SS_DOUBLE','ByteLayout',0,'Factor',1,'Offset',0,'Min',0,'Max',255,'SgnComment',{{}},'SgnUnit',''),'MsgIdNumFormat',0,'MsgComment',{{''}}),'Version',1.2,'general',struct('isFromLib',1)),'GroupId',struct('Group',{{'RTICAN'}},'No',1,'Behavior',{{'NAMECHANGE'}},'BlockType',{{'SINK'}},'NameChangeFlag',0),'SFcnRTICANMessage',struct('MsgType','TX','MsgName',['TX Message'],'MsgIdFormat','STD','MsgId',100,'MsgLength',2,'NumSignals',1,'SampleTime',-1,'StartTime',struct('Selected','no','Value',0),'AutoRepeatTime',struct('Selected','no','Value',0.1),'Timeout',struct('Selected','no','Value',0.1),'DelayTime',struct('Selected','no','Value',0.1),'Signal',struct('SgnName',['TX signal'],'SgnStartBit',0,'SgnLength',8,'SgnType','standard','ModeValue',-1,'DataType',['unsigned int'],'ByteLayout',['little endian'],'SLDataType','SS_DOUBLE','Factor',1,'Offset',0),'StatusSelected','yes','TimeSelected','yes','DeltaTimeSelected','yes','DelayTimeSelected','yes','EnablePortSelected','no','EnableMsgLoopback','no','DelayTimeTXCommandSelected','no','EncodeSetUnusedBitsToOne','no','UserCoding',struct('Selected','no','InterfaceFile','UserDecodingFile','FcnName','UserDecodeFcn','InportSelected','no','InportWidth',1,'OutportSelected','no','OutportWidth',1),'TerminationMsg',struct('Selected','no','Byte0','0x00','Byte1','0x00','Byte2','0x00','Byte3','0x00','Byte4','0x00','Byte5','0x00','Byte6','0x00','Byte7','0x00'),'InitialMsg',struct('Selected','no','Byte0','0x00','Byte1','0x00','Byte2','0x00','Byte3','0x00','Byte4','0x00','Byte5','0x00','Byte6','0x00','Byte7','0x00'),'TriggerPort',struct('Selected','no','TriggerType','rising'),'BoardType','DS4302','BoardNo',1,'ControllerNo',1,'SFcnPortType','Scalar'),'TLCFileName','rtican_tx_message')
      settings: AttributesFormatString=Group Id: RTICAN8\n
  ShiftLeverPosition : Constant  OutDataTypeMode=double  OutDataType=fixdt(1, 16)  OutScaling=2^0  OutDataTypeStr=double
  ShiftLeverPositionV : Constant  Value=0  OutDataTypeMode=double  OutDataType=fixdt(1, 16)  OutScaling=2^0  OutDataTypeStr=double
  Terminator{,1..6} (7 alike) : Terminator
  Validity{,1..5} (6 alike) : Constant  Value=0  OutDataType=fixdt(1, 16)  OutScaling=2^0
  wires:
  High_Voltage_Charger_Data_HV/1 -> Terminator/1
  ChrgrPmpPrcntSpd/1 -> High_Voltage_Charger_Data_HV/1
  ACInputCrntV/1 -> High_Voltage_Charger_Data_HV/6
  ACInputCrntV1/1 -> High_Voltage_Charger_Data_HV/7
  ACInputCrntV2/1 -> High_Voltage_Charger_Data_HV/8
  ACInputCrntV3/1 -> High_Voltage_Charger_Data_HV/9
  HVChrgLV1/1 -> High_Voltage_Charger_info_2_HV/2
  HVChrgLV/1 -> High_Voltage_Charger_info_2_HV/1
  HVChrgLV2/1 -> High_Voltage_Charger_info_2_HV/3
  HVChrgLV3/1 -> High_Voltage_Charger_info_2_HV/4
  High_Voltage_Charger_info_2_HV/1 -> Terminator1/1
  ShiftLeverPosition/1 -> PPEI_Trans_General_Status_2/16
  ShiftLeverPositionV/1 -> PPEI_Trans_General_Status_2/17
  ChargeFlashStat/1 -> High_Voltage_Charger_Data_HV/2
  Validity/1 -> High_Voltage_Charger_Out_Data_HV/1
  Validity1/1 -> High_Voltage_Charger_Out_Data_HV/2
  Validity2/1 -> High_Voltage_Charger_Out_Data_HV/3
  Validity3/1 -> High_Voltage_Charger_Out_Data_HV/4
  Validity4/1 -> High_Voltage_Charger_Out_Data_HV/5
  Validity5/1 -> High_Voltage_Charger_Out_Data_HV/6
  HVCD_ACInputTemp/1 -> Terminator2/1
  HVCD_ACInputCurr/1 -> Terminator4/1
  ChrgReadStat2/1 -> High_Voltage_Charger_Data_HV/3
  Current/1 -> High_Voltage_Charger_Data_HV/5, [Current]
  [Current] -> High_Voltage_Charger_Out_Data_HV/8
  High_Voltage_Charger_Out_Data_HV/1 -> Terminator5/1
  PPEI_Trans_General_Status_2/1 -> Terminator6/1
  Voltage/1 -> High_Voltage_Charger_Out_Data_HV/7
  ChrgReadStat3/1 -> High_Voltage_Charger_Data_HV/4
  HVCD_ACInputVltg/1 -> Terminator3/1

== system HIL_Testing_SW_amantest/LionsHeart/Calibrations/convert_CellToPack ==
  In1 : Inport  OutDataType=fixdt(1, 16)  OutScaling=2^0
  Data Store Read2 : DataStoreRead  DataStoreName=NumberOfCells  SampleTime=-1
  Divide2 : Product  Inputs=**  OutDataType=sfix(16)  OutScaling=2^-10
  Out1 : Outport  OutDataType=fixdt(1, 16)  OutScaling=2^0
  wires:
  Data Store Read2/1 -> Divide2/2
  In1/1 -> Divide2/1
  Divide2/1 -> Out1/1

== system HIL_Testing_SW_amantest/LionsHeart/Command/CS_Mode ==
  SOC : Inport  OutDataType=fixdt(1, 16)  OutScaling=2^0
  CSModeSwitch : Switch  Threshold=0.5  OutDataType=fixdt(1, 16)  OutScaling=2^0
  Data Store Read : DataStoreRead  DataStoreName=SOC_CDCS  SampleTime=0
  Data Store Read1 : DataStoreRead  DataStoreName=CSDisable  SampleTime=0
  FliptoCSMode : Constant  Value=0  OutDataTypeMode=boolean  OutDataType=sfix(16)  OutScaling=2^0  OutDataTypeStr=boolean
  Relational Operator : RelationalOperator  Operator=<=  LogicOutDataTypeMode=boolean  OutDataTypeStr=boolean
  SwitchMode : Outport  OutDataType=fixdt(1, 16)  OutScaling=2^0
  wires:
  FliptoCSMode/1 -> CSModeSwitch/1
  [CSMode] -> CSModeSwitch/3
  SOC/1 -> Relational Operator/1
  Relational Operator/1 -> [CSMode]
  CSModeSwitch/1 -> SwitchMode/1
  Data Store Read/1 -> Relational Operator/2
  Data Store Read1/1 -> CSModeSwitch/2

== system HIL_Testing_SW_amantest/LionsHeart/Command/Charge_Select ==
  ChargeCurrSelect : Inport  OutDataType=fixdt(1, 16)  OutScaling=2^0
  ManualMode : Inport  Port=2  OutDataType=fixdt(1, 16)  OutScaling=2^0
  ChargeSelect : Constant  Value=single(0)  OutDataType=sfix(16)  OutScaling=2^0
  DriveSelect1 : Switch  Threshold=0.5  OutDataType=fixdt(1, 16)  OutScaling=2^0
  Unit Delay7 : UnitDelay  SampleTime=-1
  ChargeCurrSelect_F : Outport  OutDataType=fixdt(1, 16)  OutScaling=2^0
  wires:
  ChargeSelect/1 -> DriveSelect1/1
  DriveSelect1/1 -> ChargeCurrSelect_F/1
  Unit Delay7/1 -> DriveSelect1/3
  ManualMode/1 -> DriveSelect1/2
  ChargeCurrSelect/1 -> Unit Delay7/1

== system HIL_Testing_SW_amantest/LionsHeart/Command/Drive_Select ==
  Script_Pwr : Inport  OutDataType=fixdt(1, 16)  OutScaling=2^0
  ManualMode : Inport  Port=2  OutDataType=fixdt(1, 16)  OutScaling=2^0
  DriveProfile : Constant  Value=single(0)  OutDataType=sfix(16)  OutScaling=2^0
  DriveSelect : Switch  Threshold=0.5  OutDataType=fixdt(1, 16)  OutScaling=2^0
  Unit Delay3 : UnitDelay  SampleTime=-1
  PwrCycle : Outport  OutDataType=fixdt(1, 16)  OutScaling=2^0
  wires:
  DriveProfile/1 -> DriveSelect/1
  DriveSelect/1 -> PwrCycle/1
  Script_Pwr/1 -> Unit Delay3/1
  ManualMode/1 -> DriveSelect/2
  Unit Delay3/1 -> DriveSelect/3

== system HIL_Testing_SW_amantest/LionsHeart/Command/Indicator_Select ==
  Indicator_SF : Inport  OutDataType=fixdt(1, 16)  OutScaling=2^0
  ManualMode : Inport  Port=2  OutDataType=fixdt(1, 16)  OutScaling=2^0
  Profile_or_Charge_StandbySelector : Constant  Value=single(2)  OutDataType=sfix(16)  OutScaling=2^0
  Unit Delay6 : UnitDelay  SampleTime=-1
  manualMode : Switch  Threshold=0.5  OutDataType=fixdt(1, 16)  OutScaling=2^0
  Indicator : Outport  OutDataType=fixdt(1, 16)  OutScaling=2^0
  wires:
  Profile_or_Charge_StandbySelector/1 -> manualMode/1
  manualMode/1 -> Indicator/1
  Indicator_SF/1 -> Unit Delay6/1
  Unit Delay6/1 -> manualMode/3
  ManualMode/1 -> manualMode/2

== system HIL_Testing_SW_amantest/LionsHeart/Command/SOC_Select ==
  Data Store Read7 : DataStoreRead  DataStoreName=SOC  SampleTime=0
  Data Store Read8 : DataStoreRead  DataStoreName=SOC_BSE  SampleTime=0
  Gain3 : Gain  Gain=100  ParameterDataType=sfix(16)  ParameterScaling=2^0  OutDataType=sfix(16)  OutScaling=2^0
  SOC_switch : Switch  Threshold=0.5  OutDataType=fixdt(1, 16)  OutScaling=2^0
  UseBSESOC : Constant  Value=0  OutDataType=fixdt(1, 16)  OutScaling=2^0
  SOC : Outport  OutDataType=fixdt(1, 16)  OutScaling=2^0
  wires:
  Data Store Read7/1 -> Gain3/1
  Data Store Read8/1 -> SOC_switch/1
  UseBSESOC/1 -> SOC_switch/2
  Gain3/1 -> SOC_switch/3
  SOC_switch/1 -> SOC/1

== system HIL_Testing_SW_amantest/LionsHeart/FeaturePresentation/Ahr_Integration ==
  CyclerVoltage : Inport  OutDataType=fixdt(1, 16)  OutScaling=2^0
  BatTemp : Inport  Port=2  OutDataType=fixdt(1, 16)  OutScaling=2^0
  ClearAhr : Inport  Port=3  OutDataType=fixdt(1, 16)  OutScaling=2^0
  ResetSOC : Inport  Port=4  OutDataType=fixdt(1, 16)  OutScaling=2^0
  PackCurrent : Inport  Port=5  OutDataType=fixdt(1, 16)  OutScaling=2^0
  CyclerCurrent : Inport  Port=6  OutDataType=fixdt(1, 16)  OutScaling=2^0
  PackVoltage : Inport  Port=7  OutDataType=fixdt(1, 16)  OutScaling=2^0
  OCVReset : Inport  Port=8  OutDataType=fixdt(1, 16)  OutScaling=2^0
  Clear Ahr : Subsystem  Tag=x.x
      mask Type: Subsystem
      mask Display:
      | text(.52,.01,char(get_param(gcb,'Tag') ), 'horizontalAlignment','center','verticalAlignment','bottom' )
      | disp(get_param(gcb,'Name'))
  Constant : Constant  OutDataType=fixdt(1, 16)  OutScaling=2^0
  Constant1 : Constant  OutDataType=fixdt(1, 16)  OutScaling=2^0
  Cycler_Ahr : Subsystem
  Data Store Write : DataStoreWrite  DataStoreName=SOC  SampleTime=-1
  Data Store Write1 : DataStoreWrite  DataStoreName=Ahr  SampleTime=-1
  Data Store Write2 : DataStoreWrite  DataStoreName=Whr  SampleTime=-1
  Data Type Conversion : DataTypeConversion  OutDataType=sfix(16)  OutScaling=2^0
  Lookup_SOC : Subsystem  Tag=x.x
      mask Type: Subsystem
      mask Display:
      | text(.52,.01,char(get_param(gcb,'Tag') ), 'horizontalAlignment','center','verticalAlignment','bottom' )
      | disp(get_param(gcb,'Name'))
  Pack_Ahr : Subsystem
  Switch : Switch  Threshold=.5  OutDataType=fixdt(1, 16)  OutScaling=2^0
  Switch1 : Switch  Threshold=.5  OutDataType=fixdt(1, 16)  OutScaling=2^0
  wires:
  ClearAhr/1 -> Data Type Conversion/1
  Switch/1 -> Clear Ahr/Enable
  Data Type Conversion/1 -> Switch/3
  Constant/1 -> Switch/1
  [SOCReset] -> Switch/2
  [Voltage] -> Lookup_SOC/1(Voltage)
  [PackVoltage] -> Lookup_SOC/3(PackVoltage)
  [Voltage] -> Cycler_Ahr/2(Voltage)
  [PackVoltage] -> Pack_Ahr/2(PackVoltage)
  Constant1/1 -> Switch1/1
  Switch1/1 -> Lookup_SOC/Enable
  [SOCReset] -> Switch1/2
  ResetSOC/1 -> [SOCReset]
  CyclerVoltage/1 -> [Voltage]
  PackVoltage/1 -> [PackVoltage]
  OCVReset/1 -> Switch1/3
  PackCurrent/1 -> Pack_Ahr/1(PackCurrent)
  CyclerCurrent/1 -> Cycler_Ahr/1(Current)
  BatTemp/1 -> Lookup_SOC/2(BatTemp)
  Cycler_Ahr/1(SOC) -> Data Store Write/1
  Cycler_Ahr/2(Ahr) -> Data Store Write1/1
  Cycler_Ahr/3(Whr) -> Data Store Write2/1
